simulink model "slid_tst_"  (R2017a)
settings: Solver=ode45  StartTime=0.0  StopTime=15  FixedStep=.01  MaxStep=1e-2  RelTol=1e-3  EnableMultiTasking=on
values from neighbouring files (symbols this model uses):
  c = 0    [phase00_.m]
  doHyp = 1    [phaseH_.m]    (also in phaseO_.m = 0)
  kHip2 = kHip(2)    [startDemo_.m]
  kOsc1 = kOsc(1)    [startDemo_.m]
  kOsc2 = kOsc(2)    [startDemo_.m]
undefined symbols (not defined in the file or in its folder): kHip1
libraries: cstblocks x1
settings Model: Creator=Zbigniew  LastModifiedBy=Zbigniew
settings DataIOCC: LimitDataPoints=on  SaveFormat=Array  SignalLoggingSaveFormat=ModelDataLogs
settings OptimizationCC: BlockReduction=off  BooleanDataType=off
settings DebuggingCC: SaveWithParameterizedLinksMsg=none  UnderspecifiedInitializationDetection=Classic  MergeDetectMultiDrivingBlocksExec=none  SignalResolutionControl=TryResolveAllWithWarning  MultiTaskDSMMsg=warning  MultiTaskCondExecSysMsg=none
settings HardwareCC: TargetUnknown=on
settings ModelReferenceCC: PropagateSignalLabelsOutOfModel=off
settings GRTTargetCC: TargetLangStandard=C89/C90 (ANSI)  CombineOutputUpdateFcns=off  GRTInterface=on
settings ConfigComp: CovMetricSettings=dw  CovHtmlReporting=on  CovSaveCumulativeToWorkspaceVar=on  CovSaveSingleToWorkspaceVar=on  CovExternalEMLEnable=off

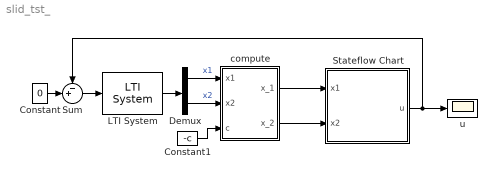
== system slid_tst_ ==
  Constant : Constant  Value=0
  Constant1 : Constant  Value=-c
  Demux : Demux  Outputs=2
  LTI System : cstblocks/LTI System  sys=sysTST  IC=ic
  Stateflow Chart : Stateflow chart  TreatAsAtomicUnit=on
  Sum : Sum  Inputs=-+|  SaturateOnIntegerOverflow=on  InputSameDT=on  OutDataTypeStr=Inherit: Same as first input
  compute : Subsystem
  u : Scope
  wires:
  Sum/1 -> LTI System/1
  Constant/1 -> Sum/2
  LTI System/1 -> Demux/1
  Demux/1 -> compute/1(x1)  "x1"
  Demux/2 -> compute/2(x2)  "x2"
  Stateflow Chart/1(u) -> Sum/1, u/1
  Constant1/1 -> compute/3(c)
  compute/1(x_1) -> Stateflow Chart/1(x1)
  compute/2(x_2) -> Stateflow Chart/2(x2)

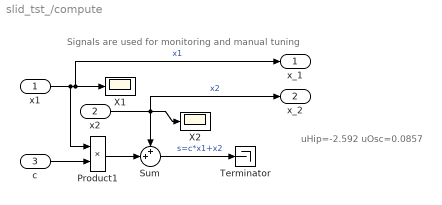
== system slid_tst_/compute ==
  note: Signals are used for monitoring and manual tuning
  note: uHip=-2.592
      | uOsc=0.0857
  x1 : Inport
  x2 : Inport  Port=2
  c : Inport  Port=3
  Product1 : Product  SaturateOnIntegerOverflow=on  RndMeth=Zero  InputSameDT=on  OutDataTypeStr=Inherit: Same as first input
  Sum : Sum  Inputs=++|  SaturateOnIntegerOverflow=on  InputSameDT=on  OutDataTypeStr=Inherit: Same as first input
  Terminator : Terminator
  X1 : Scope
  X2 : Scope
  x_1 : Outport
  x_2 : Outport  Port=2
  wires:
  x2/1 -> X2/1, Sum/1, x_2/1  "x2"
  x1/1 -> Product1/1, X1/1, x_1/1  "x1"
  Sum/1 -> Terminator/1  "s=c*x1+x2"
  Product1/1 -> Sum/2
  c/1 -> Product1/2

== stateflow chart slid_tst_/Stateflow Chart ==
  state osc/
    during:u=x1*kOsc1+x2*kOsc2;
  state hyperbolic/
    during:u=x1*kHip1+x2*kHip2;
  (default) -> osc
  osc -> hyperbolic : [doHyp==1]
  hyperbolic -> osc : [doHyp==0]
  data: x1 input double; u output double; x2 input double; doHyp local double; kHip1 parameter double; kHip2 parameter double; kOsc1 parameter double; kOsc2 parameter double
